simulink model "Project1_shaft"  (R2024b)
settings: Solver=ode1  StartTime=0.0  StopTime=10.0  FixedStep=0.02  RelTol=1e-3
values from neighbouring files (symbols this model uses):
  b = 1    [Project1_Part1.m]
  const_torque = 1    [MEEN432_Project1_Part2.m]    (also in Project1_Part1.m)
  J = 1    [Project1_Part1.m]
  omega0 = 0    [MEEN432_Project1_Part2.m]    (also in Project1_Part1.m)
  theta0 = 0    [MEEN432_Project1_Part2.m]    (also in Project1_Part1.m)
settings Model: Creator=sgopalswamy  LastModifiedBy=jpalm
settings SolverCC: AlgebraicLoopSolver=TrustRegion
settings DataIOCC: ReturnWorkspaceOutputs=off
settings DebuggingCC: UnconnectedInputMsg=warning  UnconnectedOutputMsg=warning  UnconnectedLineMsg=warning  ArithmeticOperatorsInVariantConditions=warning
settings ModelReferenceCC: EnableRefExpFcnMdlSchedulingChecks=on
settings SFSimCC: SimUseLocalCustomCode=off  CustomCodeUndefinedFunction=UseInterfaceOnly
settings RTWCC: RTWUseLocalCustomCode=off  GPUComputeCapability=3.5
settings CodeAppCC: StateflowObjectComments=on

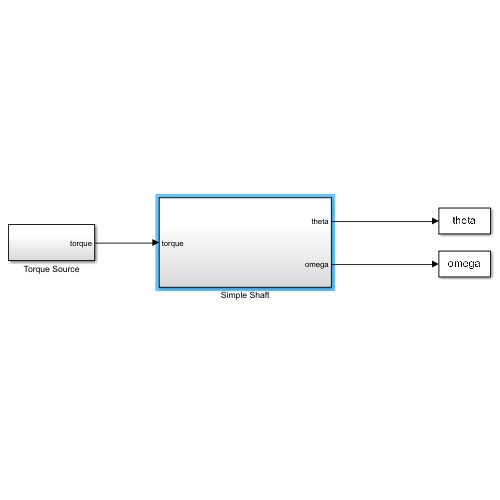
[thumbnail: Simulink's stored preview of the top-level diagram]
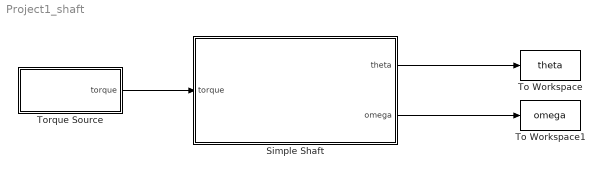
== system Project1_shaft ==
  Simple Shaft : Subsystem
  To Workspace : ToWorkspace  VariableName=theta  SaveFormat=Timeseries  SampleTime=-1
  To Workspace1 : ToWorkspace  VariableName=omega  SaveFormat=Timeseries  SampleTime=-1
  Torque Source : Subsystem
  wires:
  Torque Source/1(torque) -> Simple Shaft/1(torque)
  Simple Shaft/1(theta) -> To Workspace/1
  Simple Shaft/2(omega) -> To Workspace1/1

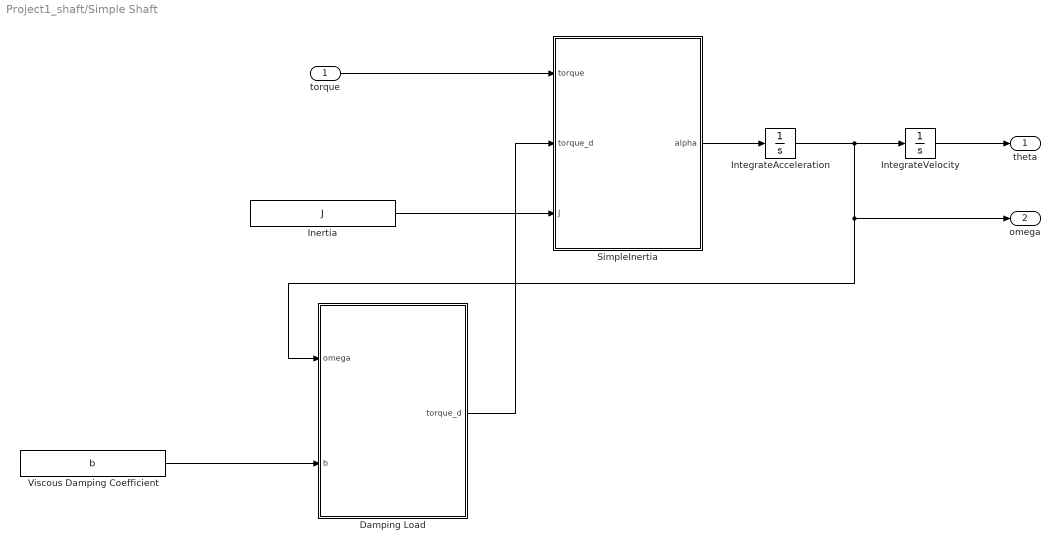
== system Project1_shaft/Simple Shaft ==
  torque : Inport
  Damping Load : MATLAB Function  TreatAsAtomicUnit=on
  Inertia : Constant  Value=J
  IntegrateAcceleration : Integrator  InitialCondition=omega0
  IntegrateVelocity : Integrator  InitialCondition=theta0
  SimpleInertia : MATLAB Function  TreatAsAtomicUnit=on
  Viscous Damping Coefficient : Constant  Value=b
  theta : Outport
  omega : Outport  Port=2
  wires:
  IntegrateAcceleration/1 -> Damping Load/1(omega), omega/1, IntegrateVelocity/1
  IntegrateVelocity/1 -> theta/1
  SimpleInertia/1(alpha) -> IntegrateAcceleration/1
  torque/1 -> SimpleInertia/1(torque)
  Viscous Damping Coefficient/1 -> Damping Load/2(b)
  Inertia/1 -> SimpleInertia/3(J)
  Damping Load/1(torque_d) -> SimpleInertia/2(torque_d)

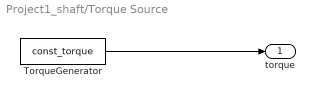
== system Project1_shaft/Torque Source ==
  TorqueGenerator : Constant  Value=const_torque
  torque : Outport
  wires:
  TorqueGenerator/1 -> torque/1

== matlab function Project1_shaft/Simple Shaft/Damping Load ==
  data: omega input; torque_d output; b input
function torque_d = fcn(omega, b)
torque_d = (omega * b);

== matlab function Project1_shaft/Simple Shaft/SimpleInertia ==
  data: torque input; torque_d input; alpha output; J input
function alpha = fcn(torque, torque_d, J)
alpha = (torque - torque_d)/J;
